simulink model "altitude_pitch_loop"  (R2016a)
settings: Solver=VariableStepAuto  StartTime=0.0  StopTime=50  RelTol=1e-3
values from neighbouring files (symbols this model uses):
  altitude_ki = wn_altitude^2 / (K_theta_DC * Va)    (= 0.0274782906556)    [tune_altitude_pitch.m]
  altitude_kp = 2 * zeta_altitude * wn_altitude / (K_theta_DC * Va)    (= 0.108310172076)    [tune_altitude_pitch.m]
  K_theta_DC = 0.4591    [tune_altitude_pitch.m]
  Va = 10    [tune_altitude_pitch.m]
settings Model: Creator=andreanv  LastModifiedBy=andreanv

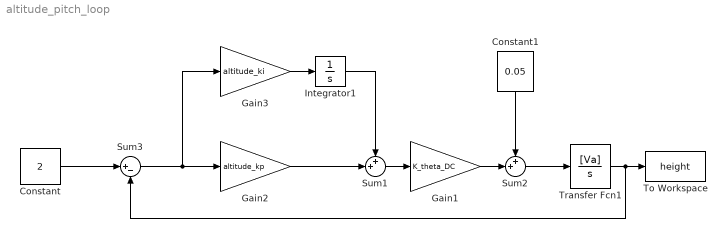
== system altitude_pitch_loop ==
  Constant : Constant  Value=2
  Constant1 : Constant  Value=0.05
  Gain1 : Gain  Gain=K_theta_DC
  Gain2 : Gain  Gain=altitude_kp
  Gain3 : Gain  Gain=altitude_ki
  Integrator1 : Integrator
  Sum1 : Sum  Inputs=++|
  Sum2 : Sum  Inputs=++|
  Sum3 : Sum  Inputs=|+-
  To Workspace : ToWorkspace  VariableName=height  SaveFormat=Timeseries  SampleTime=-1
  Transfer Fcn1 : TransferFcn  Numerator=[Va]  Denominator=[1 0]
  wires:
  Sum1/1 -> Gain1/1
  Sum2/1 -> Transfer Fcn1/1
  Transfer Fcn1/1 -> Sum3/2, To Workspace/1
  Gain2/1 -> Sum1/2
  Gain3/1 -> Integrator1/1
  Integrator1/1 -> Sum1/1
  Constant/1 -> Sum3/1
  Sum3/1 -> Gain3/1, Gain2/1
  Gain1/1 -> Sum2/2
  Constant1/1 -> Sum2/1
